simulink model "teste_hibrido_5_2"  (R2020a)
settings: Solver=VariableStepAuto  StartTime=0.0  StopTime=10.0  RelTol=1e-3
settings Model: Creator=josem  LastModifiedBy=josem

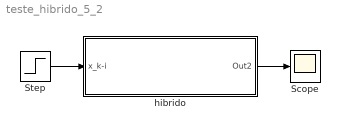
== system teste_hibrido_5_2 ==
  Scope : Scope
  Step : Step  Time=2  SampleTime=0
  hibrido : Subsystem
  wires:
  Step/1 -> hibrido/1(x_k-i)
  hibrido/1(Out2) -> Scope/1

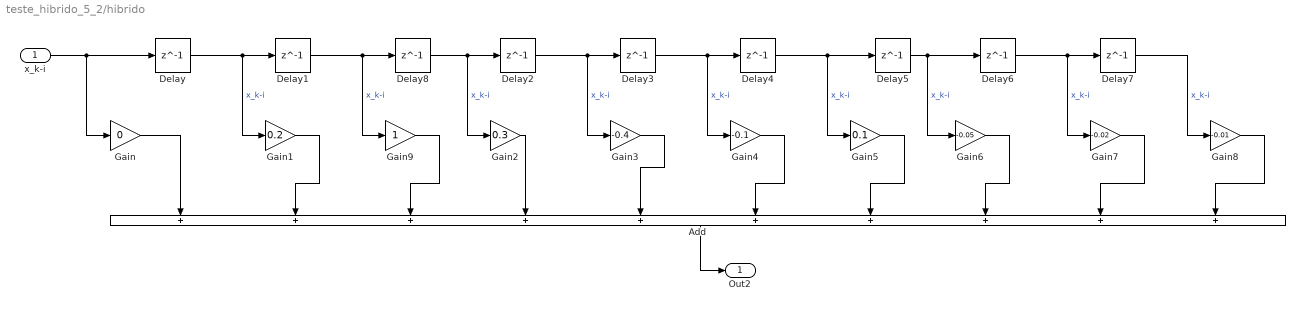
== system teste_hibrido_5_2/hibrido ==
  x_k-i : Inport
  Add : Sum  Inputs=++++++++++
  Delay{,1..8} (9 alike) : Delay  DelayLength=1  InitialCondition=0
  Gain : Gain  Gain=0
  Gain1 : Gain  Gain=0.2
  Gain2 : Gain  Gain=0.3
  Gain3 : Gain  Gain=-0.4
  Gain4 : Gain  Gain=-0.1
  Gain5 : Gain  Gain=0.1
  Gain6 : Gain  Gain=-0.05
  Gain7 : Gain  Gain=-0.02
  Gain8 : Gain  Gain=-0.01
  Gain9 : Gain
  Out2 : Outport
  wires:
  Delay6/1 -> Gain7/1, Delay7/1  "x_k-i"
  Delay5/1 -> Delay6/1, Gain6/1  "x_k-i"
  Delay3/1 -> Gain4/1, Delay4/1  "x_k-i"
  Delay7/1 -> Gain8/1  "x_k-i"
  Delay8/1 -> Gain2/1, Delay2/1  "x_k-i"
  Delay2/1 -> Gain3/1, Delay3/1  "x_k-i"
  Delay/1 -> Gain1/1, Delay1/1  "x_k-i"
  Delay4/1 -> Gain5/1, Delay5/1  "x_k-i"
  Add/1 -> Out2/1
  x_k-i/1 -> Gain/1, Delay/1
  Delay1/1 -> Gain9/1, Delay8/1  "x_k-i"
  Gain/1 -> Add/1
  Gain1/1 -> Add/2
  Gain9/1 -> Add/3
  Gain2/1 -> Add/4
  Gain3/1 -> Add/5
  Gain4/1 -> Add/6
  Gain5/1 -> Add/7
  Gain6/1 -> Add/8
  Gain7/1 -> Add/9
  Gain8/1 -> Add/10
